simulink model "CicloCompra"  (R2024b)
settings: Solver=VariableStepAuto  StartTime=0.0  StopTime=Inf  RelTol=1e-3

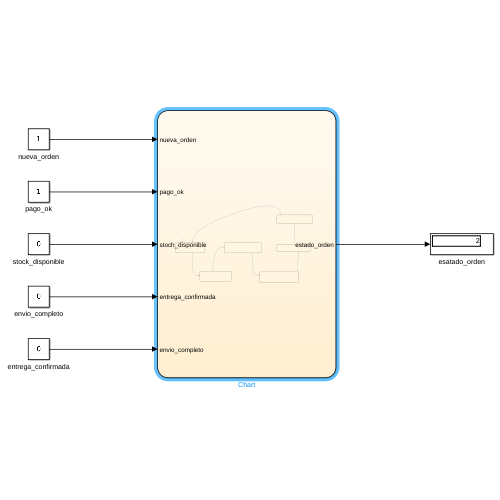
[thumbnail: Simulink's stored preview of the top-level diagram]
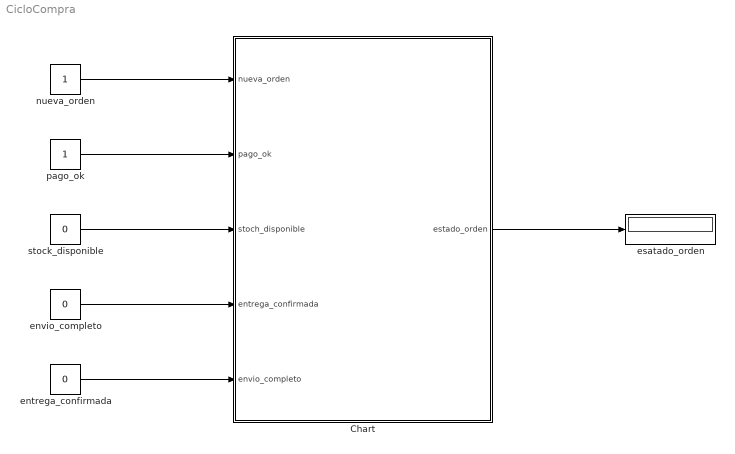
== system CicloCompra ==
  Chart : Stateflow chart  TreatAsAtomicUnit=on
  entrega_confirmada : Constant  Value=0
  envio_completo : Constant  Value=0
  esatado_orden : Display
  nueva_orden : Constant
  pago_ok : Constant
  stock_disponible : Constant  Value=0
  wires:
  Chart/1(estado_orden) -> esatado_orden/1
  nueva_orden/1 -> Chart/1(nueva_orden)
  pago_ok/1 -> Chart/2(pago_ok)
  stock_disponible/1 -> Chart/3(stoch_disponible)
  envio_completo/1 -> Chart/4(entrega_confirmada)
  entrega_confirmada/1 -> Chart/5(envio_completo)

== stateflow chart CicloCompra/Chart ==
  state Orden_Entregada
    entry:
    estado_orden=5
  state Inactivo
    entry:
    estado_orden=0
  state Pago_Verificado
    entry:
    estado_orden=2
  state Orden_Enviada
    entry:
    estado_orden=4
  state Recibida
    entry:
    estado_orden=1
  state Inventario_Asignado
    entry:
    estado_orden=3
  Orden_Entregada -> Inactivo : [after(5,sec)]
  Orden_Enviada -> Orden_Entregada : [entrega_confirmada==1]
  (default) -> Inactivo
  Recibida -> Pago_Verificado : [pago_ok==1]
  Inventario_Asignado -> Orden_Enviada : [envio_completo==1]
  Inactivo -> Recibida : [nueva_orden==1]
  Pago_Verificado -> Inventario_Asignado : [stoch_disponible==1]
  data: nueva_orden input; pago_ok input; stoch_disponible input; entrega_confirmada input; envio_completo input; estado_orden output
